simulink model "PV_MPPT_v2"  (R2025a)
settings: Solver=ode4  StartTime=0.0  StopTime=8  FixedStep=1e-5  RelTol=1e-3
model workspace (MAT data in the model file):
  MPPT_D_init = 0.5656125
  MPPT_D_max = 0.9
  MPPT_D_min = 0.05
  MPPT_D_step = 0.0005
  MPPT_P_init = 9591.75
  MPPT_Ts = 0.002
  MPPT_dP_threshold = 0.1
settings Model: Creator=Limingyu  LastModifiedBy=Limingyu
settings DataIOCC: SignalLogging=off

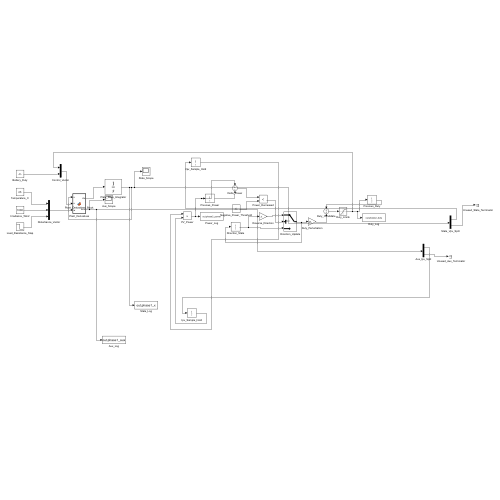
[thumbnail: Simulink's stored preview of the top-level diagram]
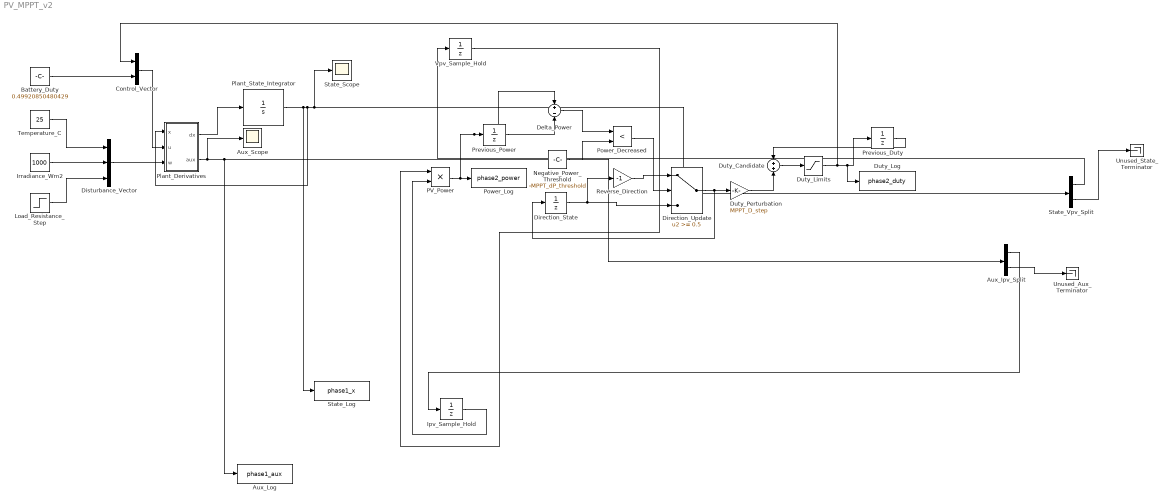
== system PV_MPPT_v2 ==
  Aux_Ipv_Split : Demux  Outputs=[1 9]
  Aux_Log : ToWorkspace  VariableName=phase1_aux  SaveFormat=Timeseries
      settings: MaxDataPoints=20000  Decimation=100
  Aux_Scope : Scope
  Battery_Duty : Constant  Value=0.49920850480429
  Control_Vector : Mux  Inputs=2
  Delta_Power : Sum  Inputs=+-
  Direction_State : UnitDelay  InitialCondition=1  SampleTime=MPPT_Ts
  Direction_Update : Switch  Threshold=0.5
  Disturbance_Vector : Mux  Inputs=3
  Duty_Candidate : Sum
  Duty_Limits : Saturate  UpperLimit=MPPT_D_max  LowerLimit=MPPT_D_min
  Duty_Log : ToWorkspace  VariableName=phase2_duty  SaveFormat=Timeseries  SampleTime=-1
  Duty_Perturbation : Gain  Gain=MPPT_D_step
  Ipv_Sample_Hold : UnitDelay  InitialCondition=36.75  SampleTime=MPPT_Ts
  Irradiance_Wm2 : Constant  Value=1000
  Load_Resistance_Step : Step  Time=4  Before=50  After=25  SampleTime=0
  Negative_Power_Threshold : Constant  Value=-MPPT_dP_threshold
  PV_Power : Product
  Plant_Derivatives : MATLAB Function  TreatAsAtomicUnit=on
  Plant_State_Integrator : Integrator  InitialCondition=[261;36.75;300.395747597855;-7.91495195710325;0.8;600]
  Power_Decreased : RelationalOperator  Operator=<
  Power_Log : ToWorkspace  VariableName=phase2_power  SaveFormat=Timeseries  SampleTime=-1
  Previous_Duty : UnitDelay  InitialCondition=MPPT_D_init  SampleTime=MPPT_Ts
  Previous_Power : UnitDelay  InitialCondition=MPPT_P_init  SampleTime=MPPT_Ts
  Reverse_Direction : Gain  Gain=-1
  State_Log : ToWorkspace  VariableName=phase1_x  SaveFormat=Timeseries
      settings: MaxDataPoints=20000  Decimation=100
  State_Scope : Scope
  State_Vpv_Split : Demux  Outputs=[1 5]
  Temperature_C : Constant  Value=25
  Unused_Aux_Terminator : Terminator
  Unused_State_Terminator : Terminator
  Vpv_Sample_Hold : UnitDelay  InitialCondition=261  SampleTime=MPPT_Ts
  wires:
  Plant_Derivatives/2(aux) -> Aux_Log/1, Aux_Ipv_Split/1, Aux_Scope/1
  Plant_State_Integrator/1 -> State_Scope/1, State_Vpv_Split/1, Plant_Derivatives/1(x), State_Log/1
  Load_Resistance_Step/1 -> Disturbance_Vector/3
  Plant_Derivatives/1(dx) -> Plant_State_Integrator/1
  Irradiance_Wm2/1 -> Disturbance_Vector/2
  Temperature_C/1 -> Disturbance_Vector/1
  Disturbance_Vector/1 -> Plant_Derivatives/3(w)
  Battery_Duty/1 -> Control_Vector/2
  Control_Vector/1 -> Plant_Derivatives/2(u)
  State_Vpv_Split/2 -> Unused_State_Terminator/1
  Aux_Ipv_Split/2 -> Unused_Aux_Terminator/1
  PV_Power/1 -> Previous_Power/1, Delta_Power/1, Power_Log/1
  Previous_Power/1 -> Delta_Power/2
  Delta_Power/1 -> Power_Decreased/1
  Negative_Power_Threshold/1 -> Power_Decreased/2
  Direction_State/1 -> Reverse_Direction/1, Direction_Update/3
  Reverse_Direction/1 -> Direction_Update/1
  Power_Decreased/1 -> Direction_Update/2
  Direction_Update/1 -> Direction_State/1, Duty_Perturbation/1
  Previous_Duty/1 -> Duty_Candidate/1
  Duty_Perturbation/1 -> Duty_Candidate/2
  Duty_Candidate/1 -> Duty_Limits/1
  Duty_Limits/1 -> Duty_Log/1, Previous_Duty/1, Control_Vector/1
  State_Vpv_Split/1 -> Vpv_Sample_Hold/1
  Vpv_Sample_Hold/1 -> PV_Power/1
  Aux_Ipv_Split/1 -> Ipv_Sample_Hold/1
  Ipv_Sample_Hold/1 -> PV_Power/2

== matlab function PV_MPPT_v2/Plant_Derivatives ==
  data: x input; u input; dx output; w input; aux output
function [dx, aux] = Plant_Derivatives_Block(x, u, w)
%PLANT_DERIVATIVES_BLOCK Paste-ready code for a MATLAB Function block.
%   Inputs:
%     x = [vpv; iLpv; vb; iLb; SoC; vdc]
%     u = [dpv; db]
%     w = [temperature_degC; irradiance_Wm2; Rload_ohm]
%
%   Outputs:
%     dx  = six continuous-time state derivatives
%     aux = [Ipv; Ib; Ebat; dpv; db; Ppv; PpvBus; ...
%            PbatBus; Pload; powerBalanceResidual]
%
%   Current signs:
%     Ib > 0 and PbatBus > 0 mean battery discharge.
%     Ib < 0 and PbatBus < 0 mean battery charge.
%
%#codegen

%% Published converter and DC-bus parameters
Cpv = 300e-6;
Lpv = 10e-3;
rLpv = 10e-3;

Cb = 300e-6;
Lb = 10e-3;
rLb = 10e-3;

Cdc = 1500e-6;

%% Published battery ratings and phase-1 assumptions
batteryCapacityAh = 20;
batteryNominalVoltage = 300;
batteryInternalResistance = 0.05;  % Phase-1 assumption
batteryNominalSoC = 0.8;
batteryOcvSlope = 0;               % Constant OCV in phase 1

%% Published PV-module data
moduleVmp = 29;
moduleImp = 7.35;
moduleVoc = 36.3;
moduleIsc = 7.84;

%% Phase-1 PV-array and environmental assumptions
seriesModules = 9;
parallelStrings = 5;
referenceTemperatureC = 25;
referenceIrradiance = 1000;
iscTempCoefficient = 0.0005 * moduleIsc;
vocTempCoefficient = -0.0032 * moduleVoc;
vocLogCoefficient = 2.0;
minimumIrradianceRatio = 1e-6;

currentRatioAtMpp = moduleImp / moduleIsc;
voltageRatioAtMpp = moduleVmp / moduleVoc;
curveExponent = log(1 - currentRatioAtMpp) ...
    / log(voltageRatioAtMpp);

%% Unpack states, commands, and disturbances
vpv = x(1);
iLpv = x(2);
vb = x(3);
iLb = x(4);
soc = x(5);
vdc = x(6);

dpv = min(max(u(1), 0), 1);
db = min(max(u(2), 0), 1);

temperatureC = w(1);
irradiance = max(w(2), 0);
Rload = max(w(3), 1);

%% Empirical PV I-V curve
if irradiance <= 1e-6
    Ipv = 0;
else
    temperatureOffset = temperatureC - referenceTemperatureC;
    irradianceRatio = irradiance / referenceIrradiance;

    moduleIscNow = moduleIsc ...
        + iscTempCoefficient * temperatureOffset;
    arrayIsc = parallelStrings * irradianceRatio ...
        * max(moduleIscNow, 0);

    moduleVocNow = moduleVoc ...
        + vocTempCoefficient * temperatureOffset ...
        + vocLogCoefficient ...
        * log(max(irradianceRatio, minimumIrradianceRatio));
    moduleVocNow = max(moduleVocNow, 1);
    arrayVoc = seriesModules * moduleVocNow;

    normalizedVoltage = max(vpv, 0) / arrayVoc;
    if normalizedVoltage >= 1
        Ipv = 0;
    else
        Ipv = arrayIsc ...
            * (1 - normalizedVoltage^curveExponent);
    end
end

%% Simplified phase-1 battery model
boundedSoC = min(max(soc, 0), 1);
Ebat = batteryNominalVoltage ...
    + batteryOcvSlope * (boundedSoC - batteryNominalSoC);
Ib = (Ebat - vb) / batteryInternalResistance;

%% Six-state averaged plant equations
dx = zeros(6, 1);
dx(1) = (Ipv - iLpv) / Cpv;
dx(2) = (-rLpv * iLpv + vpv ...
    - (1 - dpv) * vdc) / Lpv;
dx(3) = (Ib - iLb) / Cb;
dx(4) = (-rLb * iLb + vb ...
    - (1 - db) * vdc) / Lb;

% Corrected form of the paper's Equation (12): SoC depends on battery
% current, equivalently on Ebat - vb, not on inductor current x(4).
dx(5) = -Ib / (3600 * batteryCapacityAh);

dx(6) = ((1 - dpv) * iLpv ...
    + (1 - db) * iLb ...
    - vdc / Rload) / Cdc;

%% Diagnostic outputs
Ppv = vpv * Ipv;
PpvBus = vdc * (1 - dpv) * iLpv;
PbatBus = vdc * (1 - db) * iLb;
Pload = vdc^2 / Rload;
dcBusStoredPower = Cdc * vdc * dx(6);
powerBalanceResidual = PpvBus + PbatBus ...
    - Pload - dcBusStoredPower;

aux = zeros(10, 1);
aux(1) = Ipv;
aux(2) = Ib;
aux(3) = Ebat;
aux(4) = dpv;
aux(5) = db;
aux(6) = Ppv;
aux(7) = PpvBus;
aux(8) = PbatBus;
aux(9) = Pload;
aux(10) = powerBalanceResidual;
end
